simulink model "ES320A_MotDrvDiagc"  (R2013b)
settings: Solver=FixedStepDiscrete  StartTime=0.0  StopTime=1  FixedStep=.002  RelTol=1e-3
undefined symbols (not defined in the file): ARCHGLBPRM_2MILLISEC_SEC_F32, MotDrvDiagcErrFilFrq, MotDrvDiagcErrOffs, MotDrvDiagcErrThd, NtcNr1, NtcSts1, PHAONTISUMMAX_NANOSEC_U32, SysSt1
libraries: simulink x23, Fil x12, NxtrAbslt x6, NxtrLim x6
(part 3 of 3)

== system ES320A_MotDrvDiagc/MotDrvDiagc/MotDrvDiagcPer1/MotDrvDiagcFltChk/MeasdPhaFltChkABC/NtcStInfoPhaC/DetermineBitsetC1 ==
  Action Port : ActionPort  ActionType=else
  Constant5 : Constant  Value=0  OutDataTypeStr=uint8
  Copyright1 : Subsystem  Description=|  RequirementInfo={} %GIDa_4733e405_2a62_4416_a20f_f2380524059e  mask(Copyright Information){none=on}
      | Copyright info block.                                               
      |                                                                     
      | Place copyright information at the top of every subsystem in design.
      mask prompts: none "No parameters"
      mask help: Place copyright information at the top of every subsystem in design.
      mask Display:
      | NxtrConf = 'Nexteer Confidential';
      | 
      | sys = bdroot; %handle for the current model ("system")
      | first = get_param(sys,'Created');
      | if(isempty(first))
      |     first = datestr(now,'yyyy');
      | else
      |     first = first(end-3:end);  %year is last four digits
      | end
      | 
      | last = get_param(sys,'LastModifiedDate');
      | if isempty(last)
      |     last = datestr(now,'yyyy');
      | else
      |     last = last(end-3:end);
      | end
      | 
      | if strcmp(first,last)
      |     fprintf('%s\nCopyright  %s Nexteer',NxtrConf,first);
      | else
      |     fprintf('%s\n%s%s-%s Nexteer',NxtrConf,char(169),first,last);
      | end
  BitSetC : Outport
  wires:
  Constant5/1 -> BitSetC/1

== system ES320A_MotDrvDiagc/MotDrvDiagc/MotDrvDiagcPer1/MotDrvDiagcFltChk/MeasdPhaFltChkABC/NtcStsPhaABC/Copyright1 ==

== system ES320A_MotDrvDiagc/MotDrvDiagc/MotDrvDiagcPer1/MotDrvDiagcFltChk/MeasdPhaFltChkABC/NtcStsPhaABC/NtcFailed ==
  Action Port : ActionPort  ActionType=else
  Copyright1 : Subsystem  Description=|  RequirementInfo={} %GIDa_bd5e996a_5d08_43f2_9ecd_b972bb3ae5f6  mask(Copyright Information){none=on}
      | Copyright info block.                                               
      |                                                                     
      | Place copyright information at the top of every subsystem in design.
      mask prompts: none "No parameters"
      mask help: Place copyright information at the top of every subsystem in design.
      mask Display:
      | NxtrConf = 'Nexteer Confidential';
      | 
      | sys = bdroot; %handle for the current model ("system")
      | first = get_param(sys,'Created');
      | if(isempty(first))
      |     first = datestr(now,'yyyy');
      | else
      |     first = first(end-3:end);  %year is last four digits
      | end
      | 
      | last = get_param(sys,'LastModifiedDate');
      | if isempty(last)
      |     last = datestr(now,'yyyy');
      | else
      |     last = last(end-3:end);
      | end
      | 
      | if strcmp(first,last)
      |     fprintf('%s\nCopyright  %s Nexteer',NxtrConf,first);
      | else
      |     fprintf('%s\n%s%s-%s Nexteer',NxtrConf,char(169),first,last);
      | end
  NtcSts : simulink/Sources/Enumerated Constant  OutDataTypeStr=Enum: NtcSts1  Value=NtcSts1.NTCSTS_FAILD  SampleTime=inf
  NtcSts1 : Outport
  wires:
  NtcSts/1 -> NtcSts1/1

== system ES320A_MotDrvDiagc/MotDrvDiagc/MotDrvDiagcPer1/MotDrvDiagcFltChk/MeasdPhaFltChkABC/NtcStsPhaABC/NtcPassed ==
  Action Port : ActionPort  ActionType=then
  Copyright1 : Subsystem  Description=|  RequirementInfo={} %GIDa_99e6e5b4_d746_41cc_912e_5ec491f39e50  mask(Copyright Information){none=on}
      | Copyright info block.                                               
      |                                                                     
      | Place copyright information at the top of every subsystem in design.
      mask prompts: none "No parameters"
      mask help: Place copyright information at the top of every subsystem in design.
      mask Display:
      | NxtrConf = 'Nexteer Confidential';
      | 
      | sys = bdroot; %handle for the current model ("system")
      | first = get_param(sys,'Created');
      | if(isempty(first))
      |     first = datestr(now,'yyyy');
      | else
      |     first = first(end-3:end);  %year is last four digits
      | end
      | 
      | last = get_param(sys,'LastModifiedDate');
      | if isempty(last)
      |     last = datestr(now,'yyyy');
      | else
      |     last = last(end-3:end);
      | end
      | 
      | if strcmp(first,last)
      |     fprintf('%s\nCopyright  %s Nexteer',NxtrConf,first);
      | else
      |     fprintf('%s\n%s%s-%s Nexteer',NxtrConf,char(169),first,last);
      | end
  NtcSts : simulink/Sources/Enumerated Constant  OutDataTypeStr=Enum: NtcSts1  Value=NtcSts1.NTCSTS_PASSD  SampleTime=inf
  NtcSts1 : Outport
  wires:
  NtcSts/1 -> NtcSts1/1

== system ES320A_MotDrvDiagc/MotDrvDiagc/MotDrvDiagcPer1/MotDrvDiagcFltChk/MeasdPhaFltChkABC/SetNtcSts/Copyright1 ==

== system ES320A_MotDrvDiagc/MotDrvDiagc/MotDrvDiagcPer1/MotDrvDiagcFltChk/MeasdPhaFltChkDEF/FltLmtA/Copyright1 ==

== system ES320A_MotDrvDiagc/MotDrvDiagc/MotDrvDiagcPer1/MotDrvDiagcFltChk/MeasdPhaFltChkDEF/FltLmtB/Copyright1 ==

== system ES320A_MotDrvDiagc/MotDrvDiagc/MotDrvDiagcPer1/MotDrvDiagcFltChk/MeasdPhaFltChkDEF/FltLmtC/Copyright1 ==

== system ES320A_MotDrvDiagc/MotDrvDiagc/MotDrvDiagcPer1/MotDrvDiagcFltChk/MeasdPhaFltChkDEF/NtcStInfoPhaD/Copyright1 ==

== system ES320A_MotDrvDiagc/MotDrvDiagc/MotDrvDiagcPer1/MotDrvDiagcFltChk/MeasdPhaFltChkDEF/NtcStInfoPhaD/DetermineBitsetD ==
  PhaOnTiMeasdD : Inport
  PhaOnTiSumAExp : Inport  Port=2
  Action Port : ActionPort  ActionType=then
  BitsetStsD : Subsystem  RequirementInfo={'linktype_rmi_doors' '0000cf4c (/ESG Group/FDD Module Requirements/EA4 Specific/ES320A_MotDrvDiagc)' '#ES320A_196' 'true' 'REQ: ES320A_196' '' } %GIDa_8260d35a_8abd_420d_bbec_6159932b305c  TreatAsAtomicUnit=on
  BitsetStsD1 : Subsystem  RequirementInfo={'linktype_rmi_doors' '0000cf4c (/ESG Group/FDD Module Requirements/EA4 Specific/ES320A_MotDrvDiagc)' '#ES320A_197' 'true' 'REQ: ES320A_197' '' } %GIDa_48a41a6a_6f15_404d_a5f0_60e64f87e767  TreatAsAtomicUnit=on
  Copyright1 : Subsystem  Description=|  RequirementInfo={} %GIDa_1788af49_bd75_4060_896f_185cb50ec618  mask(Copyright Information){none=on}
      | Copyright info block.                                               
      |                                                                     
      | Place copyright information at the top of every subsystem in design.
      mask prompts: none "No parameters"
      mask help: Place copyright information at the top of every subsystem in design.
      mask Display:
      | NxtrConf = 'Nexteer Confidential';
      | 
      | sys = bdroot; %handle for the current model ("system")
      | first = get_param(sys,'Created');
      | if(isempty(first))
      |     first = datestr(now,'yyyy');
      | else
      |     first = first(end-3:end);  %year is last four digits
      | end
      | 
      | last = get_param(sys,'LastModifiedDate');
      | if isempty(last)
      |     last = datestr(now,'yyyy');
      | else
      |     last = last(end-3:end);
      | end
      | 
      | if strcmp(first,last)
      |     fprintf('%s\nCopyright  %s Nexteer',NxtrConf,first);
      | else
      |     fprintf('%s\n%s%s-%s Nexteer',NxtrConf,char(169),first,last);
      | end
  If : If  IfExpression=u1
  Merge : Merge
  Relational Operator : RelationalOperator  Operator=<  OutDataTypeStr=boolean
  BitSetD : Outport
  wires:
  BitsetStsD/1(bitsetD) -> Merge/1
  BitsetStsD1/1(bitsetD) -> Merge/2
  Merge/1 -> BitSetD/1
  If/1 -> BitsetStsD/Action
  PhaOnTiMeasdD/1 -> Relational Operator/1
  PhaOnTiSumAExp/1 -> Relational Operator/2
  If/2 -> BitsetStsD1/Action
  Relational Operator/1 -> If/1

== system ES320A_MotDrvDiagc/MotDrvDiagc/MotDrvDiagcPer1/MotDrvDiagcFltChk/MeasdPhaFltChkDEF/NtcStInfoPhaD/DetermineBitsetD1 ==
  Action Port : ActionPort  ActionType=else
  Constant5 : Constant  Value=0  OutDataTypeStr=uint8
  Copyright1 : Subsystem  Description=|  RequirementInfo={} %GIDa_7d3de8bf_4d93_4aaf_a970_cfd48355e2a0  mask(Copyright Information){none=on}
      | Copyright info block.                                               
      |                                                                     
      | Place copyright information at the top of every subsystem in design.
      mask prompts: none "No parameters"
      mask help: Place copyright information at the top of every subsystem in design.
      mask Display:
      | NxtrConf = 'Nexteer Confidential';
      | 
      | sys = bdroot; %handle for the current model ("system")
      | first = get_param(sys,'Created');
      | if(isempty(first))
      |     first = datestr(now,'yyyy');
      | else
      |     first = first(end-3:end);  %year is last four digits
      | end
      | 
      | last = get_param(sys,'LastModifiedDate');
      | if isempty(last)
      |     last = datestr(now,'yyyy');
      | else
      |     last = last(end-3:end);
      | end
      | 
      | if strcmp(first,last)
      |     fprintf('%s\nCopyright  %s Nexteer',NxtrConf,first);
      | else
      |     fprintf('%s\n%s%s-%s Nexteer',NxtrConf,char(169),first,last);
      | end
  BitSetD : Outport
  wires:
  Constant5/1 -> BitSetD/1

== system ES320A_MotDrvDiagc/MotDrvDiagc/MotDrvDiagcPer1/MotDrvDiagcFltChk/MeasdPhaFltChkDEF/NtcStInfoPhaE/Copyright1 ==

== system ES320A_MotDrvDiagc/MotDrvDiagc/MotDrvDiagcPer1/MotDrvDiagcFltChk/MeasdPhaFltChkDEF/NtcStInfoPhaE/DetermineBitsetE ==
  PhaOnTiMeasdE : Inport
  PhaOnTiSumBExp : Inport  Port=2
  Action Port : ActionPort  ActionType=then
  BitsetStsE : Subsystem  RequirementInfo={'linktype_rmi_doors' '0000cf4c (/ESG Group/FDD Module Requirements/EA4 Specific/ES320A_MotDrvDiagc)' '#ES320A_198' 'true' 'REQ: ES320A_198' '' } %GIDa_08169722_133b_47d0_8dcc_55ebdb8fb1a5  TreatAsAtomicUnit=on
  BitsetStsE1 : Subsystem  RequirementInfo={'linktype_rmi_doors' '0000cf4c (/ESG Group/FDD Module Requirements/EA4 Specific/ES320A_MotDrvDiagc)' '#ES320A_199' 'true' 'REQ: ES320A_199' '' } %GIDa_359415b0_e38b_416f_8765_3117a83da501  TreatAsAtomicUnit=on
  Copyright1 : Subsystem  Description=|  RequirementInfo={} %GIDa_7c5a11b8_a3a6_4c1e_aad7_eeec68a14235  mask(Copyright Information){none=on}
      | Copyright info block.                                               
      |                                                                     
      | Place copyright information at the top of every subsystem in design.
      mask prompts: none "No parameters"
      mask help: Place copyright information at the top of every subsystem in design.
      mask Display:
      | NxtrConf = 'Nexteer Confidential';
      | 
      | sys = bdroot; %handle for the current model ("system")
      | first = get_param(sys,'Created');
      | if(isempty(first))
      |     first = datestr(now,'yyyy');
      | else
      |     first = first(end-3:end);  %year is last four digits
      | end
      | 
      | last = get_param(sys,'LastModifiedDate');
      | if isempty(last)
      |     last = datestr(now,'yyyy');
      | else
      |     last = last(end-3:end);
      | end
      | 
      | if strcmp(first,last)
      |     fprintf('%s\nCopyright  %s Nexteer',NxtrConf,first);
      | else
      |     fprintf('%s\n%s%s-%s Nexteer',NxtrConf,char(169),first,last);
      | end
  If : If  IfExpression=u1
  Merge : Merge
  Relational Operator : RelationalOperator  Operator=<  OutDataTypeStr=boolean
  BitSetE : Outport
  wires:
  PhaOnTiSumBExp/1 -> Relational Operator/2
  PhaOnTiMeasdE/1 -> Relational Operator/1
  BitsetStsE/1(bitsetE) -> Merge/1
  BitsetStsE1/1(bitsetE) -> Merge/2
  Merge/1 -> BitSetE/1
  If/1 -> BitsetStsE/Action
  If/2 -> BitsetStsE1/Action
  Relational Operator/1 -> If/1

== system ES320A_MotDrvDiagc/MotDrvDiagc/MotDrvDiagcPer1/MotDrvDiagcFltChk/MeasdPhaFltChkDEF/NtcStInfoPhaE/DetermineBitsetE1 ==
  Action Port : ActionPort  ActionType=else
  Constant5 : Constant  Value=0  OutDataTypeStr=uint8
  Copyright1 : Subsystem  Description=|  RequirementInfo={} %GIDa_2e7c738b_8ed4_4057_8dbe_cf0f29a374b5  mask(Copyright Information){none=on}
      | Copyright info block.                                               
      |                                                                     
      | Place copyright information at the top of every subsystem in design.
      mask prompts: none "No parameters"
      mask help: Place copyright information at the top of every subsystem in design.
      mask Display:
      | NxtrConf = 'Nexteer Confidential';
      | 
      | sys = bdroot; %handle for the current model ("system")
      | first = get_param(sys,'Created');
      | if(isempty(first))
      |     first = datestr(now,'yyyy');
      | else
      |     first = first(end-3:end);  %year is last four digits
      | end
      | 
      | last = get_param(sys,'LastModifiedDate');
      | if isempty(last)
      |     last = datestr(now,'yyyy');
      | else
      |     last = last(end-3:end);
      | end
      | 
      | if strcmp(first,last)
      |     fprintf('%s\nCopyright  %s Nexteer',NxtrConf,first);
      | else
      |     fprintf('%s\n%s%s-%s Nexteer',NxtrConf,char(169),first,last);
      | end
  BitSetE : Outport
  wires:
  Constant5/1 -> BitSetE/1

== system ES320A_MotDrvDiagc/MotDrvDiagc/MotDrvDiagcPer1/MotDrvDiagcFltChk/MeasdPhaFltChkDEF/NtcStInfoPhaF/Copyright1 ==

== system ES320A_MotDrvDiagc/MotDrvDiagc/MotDrvDiagcPer1/MotDrvDiagcFltChk/MeasdPhaFltChkDEF/NtcStInfoPhaF/DetermineBitsetF ==
  PhaOnTiMeasdF : Inport
  PhaOnTiSumCExp : Inport  Port=2
  Action Port : ActionPort  ActionType=then
  BitsetStsF : Subsystem  RequirementInfo={'linktype_rmi_doors' '0000cf4c (/ESG Group/FDD Module Requirements/EA4 Specific/ES320A_MotDrvDiagc)' '#ES320A_200' 'true' 'REQ: ES320A_200' '' } %GIDa_55a58c0c_abfb_4587_b479_1d90e8aa5549  TreatAsAtomicUnit=on
  BitsetStsF1 : Subsystem  RequirementInfo={'linktype_rmi_doors' '0000cf4c (/ESG Group/FDD Module Requirements/EA4 Specific/ES320A_MotDrvDiagc)' '#ES320A_201' 'true' 'REQ: ES320A_201' '' } %GIDa_a8dfb83c_85c1_4b48_a1e1_aa37e2bdfe1a  TreatAsAtomicUnit=on
  Copyright1 : Subsystem  Description=|  RequirementInfo={} %GIDa_fb0ae897_2b05_462f_9fe8_c1b0d422596f  mask(Copyright Information){none=on}
      | Copyright info block.                                               
      |                                                                     
      | Place copyright information at the top of every subsystem in design.
      mask prompts: none "No parameters"
      mask help: Place copyright information at the top of every subsystem in design.
      mask Display:
      | NxtrConf = 'Nexteer Confidential';
      | 
      | sys = bdroot; %handle for the current model ("system")
      | first = get_param(sys,'Created');
      | if(isempty(first))
      |     first = datestr(now,'yyyy');
      | else
      |     first = first(end-3:end);  %year is last four digits
      | end
      | 
      | last = get_param(sys,'LastModifiedDate');
      | if isempty(last)
      |     last = datestr(now,'yyyy');
      | else
      |     last = last(end-3:end);
      | end
      | 
      | if strcmp(first,last)
      |     fprintf('%s\nCopyright  %s Nexteer',NxtrConf,first);
      | else
      |     fprintf('%s\n%s%s-%s Nexteer',NxtrConf,char(169),first,last);
      | end
  If : If  IfExpression=u1
  Merge : Merge
  Relational Operator : RelationalOperator  Operator=<  OutDataTypeStr=boolean
  BitSetF : Outport
  wires:
  BitsetStsF/1(bitsetF) -> Merge/1
  BitsetStsF1/1(bitsetF) -> Merge/2
  Merge/1 -> BitSetF/1
  PhaOnTiSumCExp/1 -> Relational Operator/2
  PhaOnTiMeasdF/1 -> Relational Operator/1
  If/1 -> BitsetStsF/Action
  If/2 -> BitsetStsF1/Action
  Relational Operator/1 -> If/1

== system ES320A_MotDrvDiagc/MotDrvDiagc/MotDrvDiagcPer1/MotDrvDiagcFltChk/MeasdPhaFltChkDEF/NtcStInfoPhaF/DetermineBitsetF1 ==
  Action Port : ActionPort  ActionType=else
  Constant5 : Constant  Value=0  OutDataTypeStr=uint8
  Copyright1 : Subsystem  Description=|  RequirementInfo={} %GIDa_d82a1e1b_c682_4f73_a346_e773759e2be9  mask(Copyright Information){none=on}
      | Copyright info block.                                               
      |                                                                     
      | Place copyright information at the top of every subsystem in design.
      mask prompts: none "No parameters"
      mask help: Place copyright information at the top of every subsystem in design.
      mask Display:
      | NxtrConf = 'Nexteer Confidential';
      | 
      | sys = bdroot; %handle for the current model ("system")
      | first = get_param(sys,'Created');
      | if(isempty(first))
      |     first = datestr(now,'yyyy');
      | else
      |     first = first(end-3:end);  %year is last four digits
      | end
      | 
      | last = get_param(sys,'LastModifiedDate');
      | if isempty(last)
      |     last = datestr(now,'yyyy');
      | else
      |     last = last(end-3:end);
      | end
      | 
      | if strcmp(first,last)
      |     fprintf('%s\nCopyright  %s Nexteer',NxtrConf,first);
      | else
      |     fprintf('%s\n%s%s-%s Nexteer',NxtrConf,char(169),first,last);
      | end
  BitSetF : Outport
  wires:
  Constant5/1 -> BitSetF/1

== system ES320A_MotDrvDiagc/MotDrvDiagc/MotDrvDiagcPer1/MotDrvDiagcFltChk/MeasdPhaFltChkDEF/NtcStsPhaDEF/Copyright1 ==

== system ES320A_MotDrvDiagc/MotDrvDiagc/MotDrvDiagcPer1/MotDrvDiagcFltChk/MeasdPhaFltChkDEF/NtcStsPhaDEF/NtcFailed ==
  Action Port : ActionPort  ActionType=else
  Copyright1 : Subsystem  Description=|  RequirementInfo={} %GIDa_17e947be_2e1f_4709_9ef4_8520ceffa1b1  mask(Copyright Information){none=on}
      | Copyright info block.                                               
      |                                                                     
      | Place copyright information at the top of every subsystem in design.
      mask prompts: none "No parameters"
      mask help: Place copyright information at the top of every subsystem in design.
      mask Display:
      | NxtrConf = 'Nexteer Confidential';
      | 
      | sys = bdroot; %handle for the current model ("system")
      | first = get_param(sys,'Created');
      | if(isempty(first))
      |     first = datestr(now,'yyyy');
      | else
      |     first = first(end-3:end);  %year is last four digits
      | end
      | 
      | last = get_param(sys,'LastModifiedDate');
      | if isempty(last)
      |     last = datestr(now,'yyyy');
      | else
      |     last = last(end-3:end);
      | end
      | 
      | if strcmp(first,last)
      |     fprintf('%s\nCopyright  %s Nexteer',NxtrConf,first);
      | else
      |     fprintf('%s\n%s%s-%s Nexteer',NxtrConf,char(169),first,last);
      | end
  NtcSts : simulink/Sources/Enumerated Constant  OutDataTypeStr=Enum: NtcSts1  Value=NtcSts1.NTCSTS_FAILD  SampleTime=inf
  NtcSts1 : Outport
  wires:
  NtcSts/1 -> NtcSts1/1

== system ES320A_MotDrvDiagc/MotDrvDiagc/MotDrvDiagcPer1/MotDrvDiagcFltChk/MeasdPhaFltChkDEF/NtcStsPhaDEF/NtcPassed ==
  Action Port : ActionPort  ActionType=then
  Copyright1 : Subsystem  Description=|  RequirementInfo={} %GIDa_1122f953_822e_40b1_bb4c_1cb6bb86ea20  mask(Copyright Information){none=on}
      | Copyright info block.                                               
      |                                                                     
      | Place copyright information at the top of every subsystem in design.
      mask prompts: none "No parameters"
      mask help: Place copyright information at the top of every subsystem in design.
      mask Display:
      | NxtrConf = 'Nexteer Confidential';
      | 
      | sys = bdroot; %handle for the current model ("system")
      | first = get_param(sys,'Created');
      | if(isempty(first))
      |     first = datestr(now,'yyyy');
      | else
      |     first = first(end-3:end);  %year is last four digits
      | end
      | 
      | last = get_param(sys,'LastModifiedDate');
      | if isempty(last)
      |     last = datestr(now,'yyyy');
      | else
      |     last = last(end-3:end);
      | end
      | 
      | if strcmp(first,last)
      |     fprintf('%s\nCopyright  %s Nexteer',NxtrConf,first);
      | else
      |     fprintf('%s\n%s%s-%s Nexteer',NxtrConf,char(169),first,last);
      | end
  NtcSts : simulink/Sources/Enumerated Constant  OutDataTypeStr=Enum: NtcSts1  Value=NtcSts1.NTCSTS_PASSD  SampleTime=inf
  NtcSts1 : Outport
  wires:
  NtcSts/1 -> NtcSts1/1

== system ES320A_MotDrvDiagc/MotDrvDiagc/MotDrvDiagcPer1/MotDrvDiagcFltChk/MeasdPhaFltChkDEF/SetNtcSts/Copyright1 ==

== system ES320A_MotDrvDiagc/MotDrvDiagc/MotDrvDiagcPer1/MotDrvDiagcFltChk/MeasdPhaFltChkABC/NtcStInfoPhaA/DetermineBitsetA/BitsetStsA ==
  Action Port : ActionPort  ActionType=then
  Bit Set : simulink/Logic and Bit Operations/Bit Set  iBit=0
  Constant : Constant  Value=0  OutDataTypeStr=uint8
  Copyright1 : Subsystem  Description=|  RequirementInfo={} %GIDa_cdd52c65_1ab2_45c6_a6fc_5222191c335e  mask(Copyright Information){none=on}
      | Copyright info block.                                               
      |                                                                     
      | Place copyright information at the top of every subsystem in design.
      mask prompts: none "No parameters"
      mask help: Place copyright information at the top of every subsystem in design.
      mask Display:
      | NxtrConf = 'Nexteer Confidential';
      | 
      | sys = bdroot; %handle for the current model ("system")
      | first = get_param(sys,'Created');
      | if(isempty(first))
      |     first = datestr(now,'yyyy');
      | else
      |     first = first(end-3:end);  %year is last four digits
      | end
      | 
      | last = get_param(sys,'LastModifiedDate');
      | if isempty(last)
      |     last = datestr(now,'yyyy');
      | else
      |     last = last(end-3:end);
      | end
      | 
      | if strcmp(first,last)
      |     fprintf('%s\nCopyright  %s Nexteer',NxtrConf,first);
      | else
      |     fprintf('%s\n%s%s-%s Nexteer',NxtrConf,char(169),first,last);
      | end
  bitsetA : Outport
  wires:
  Constant/1 -> Bit Set/1
  Bit Set/1 -> bitsetA/1

== system ES320A_MotDrvDiagc/MotDrvDiagc/MotDrvDiagcPer1/MotDrvDiagcFltChk/MeasdPhaFltChkABC/NtcStInfoPhaA/DetermineBitsetA/BitsetStsA1 ==
  Action Port : ActionPort  ActionType=else
  Bit Set1 : simulink/Logic and Bit Operations/Bit Set  iBit=1
  Constant6 : Constant  Value=0  OutDataTypeStr=uint8
  Copyright1 : Subsystem  Description=|  RequirementInfo={} %GIDa_4a3532e0_542b_44ef_af96_af0d103a28d1  mask(Copyright Information){none=on}
      | Copyright info block.                                               
      |                                                                     
      | Place copyright information at the top of every subsystem in design.
      mask prompts: none "No parameters"
      mask help: Place copyright information at the top of every subsystem in design.
      mask Display:
      | NxtrConf = 'Nexteer Confidential';
      | 
      | sys = bdroot; %handle for the current model ("system")
      | first = get_param(sys,'Created');
      | if(isempty(first))
      |     first = datestr(now,'yyyy');
      | else
      |     first = first(end-3:end);  %year is last four digits
      | end
      | 
      | last = get_param(sys,'LastModifiedDate');
      | if isempty(last)
      |     last = datestr(now,'yyyy');
      | else
      |     last = last(end-3:end);
      | end
      | 
      | if strcmp(first,last)
      |     fprintf('%s\nCopyright  %s Nexteer',NxtrConf,first);
      | else
      |     fprintf('%s\n%s%s-%s Nexteer',NxtrConf,char(169),first,last);
      | end
  bitsetA : Outport
  wires:
  Constant6/1 -> Bit Set1/1
  Bit Set1/1 -> bitsetA/1

== system ES320A_MotDrvDiagc/MotDrvDiagc/MotDrvDiagcPer1/MotDrvDiagcFltChk/MeasdPhaFltChkABC/NtcStInfoPhaA/DetermineBitsetA/Copyright1 ==

== system ES320A_MotDrvDiagc/MotDrvDiagc/MotDrvDiagcPer1/MotDrvDiagcFltChk/MeasdPhaFltChkABC/NtcStInfoPhaA/DetermineBitsetA1/Copyright1 ==

== system ES320A_MotDrvDiagc/MotDrvDiagc/MotDrvDiagcPer1/MotDrvDiagcFltChk/MeasdPhaFltChkABC/NtcStInfoPhaB/DetermineBitsetB/BitsetStsB ==
  Action Port : ActionPort  ActionType=then
  Bit Set : simulink/Logic and Bit Operations/Bit Set  iBit=2
  Constant : Constant  Value=0  OutDataTypeStr=uint8
  Copyright1 : Subsystem  Description=|  RequirementInfo={} %GIDa_c1b71190_810a_4c1f_9336_9d9ddd65ac32  mask(Copyright Information){none=on}
      | Copyright info block.                                               
      |                                                                     
      | Place copyright information at the top of every subsystem in design.
      mask prompts: none "No parameters"
      mask help: Place copyright information at the top of every subsystem in design.
      mask Display:
      | NxtrConf = 'Nexteer Confidential';
      | 
      | sys = bdroot; %handle for the current model ("system")
      | first = get_param(sys,'Created');
      | if(isempty(first))
      |     first = datestr(now,'yyyy');
      | else
      |     first = first(end-3:end);  %year is last four digits
      | end
      | 
      | last = get_param(sys,'LastModifiedDate');
      | if isempty(last)
      |     last = datestr(now,'yyyy');
      | else
      |     last = last(end-3:end);
      | end
      | 
      | if strcmp(first,last)
      |     fprintf('%s\nCopyright  %s Nexteer',NxtrConf,first);
      | else
      |     fprintf('%s\n%s%s-%s Nexteer',NxtrConf,char(169),first,last);
      | end
  bitsetB : Outport
  wires:
  Constant/1 -> Bit Set/1
  Bit Set/1 -> bitsetB/1

== system ES320A_MotDrvDiagc/MotDrvDiagc/MotDrvDiagcPer1/MotDrvDiagcFltChk/MeasdPhaFltChkABC/NtcStInfoPhaB/DetermineBitsetB/BitsetStsB1 ==
  Action Port : ActionPort  ActionType=else
  Bit Set1 : simulink/Logic and Bit Operations/Bit Set  iBit=3
  Constant6 : Constant  Value=0  OutDataTypeStr=uint8
  Copyright1 : Subsystem  Description=|  RequirementInfo={} %GIDa_1c98625e_4ddf_4d14_b0b0_5f8b66934288  mask(Copyright Information){none=on}
      | Copyright info block.                                               
      |                                                                     
      | Place copyright information at the top of every subsystem in design.
      mask prompts: none "No parameters"
      mask help: Place copyright information at the top of every subsystem in design.
      mask Display:
      | NxtrConf = 'Nexteer Confidential';
      | 
      | sys = bdroot; %handle for the current model ("system")
      | first = get_param(sys,'Created');
      | if(isempty(first))
      |     first = datestr(now,'yyyy');
      | else
      |     first = first(end-3:end);  %year is last four digits
      | end
      | 
      | last = get_param(sys,'LastModifiedDate');
      | if isempty(last)
      |     last = datestr(now,'yyyy');
      | else
      |     last = last(end-3:end);
      | end
      | 
      | if strcmp(first,last)
      |     fprintf('%s\nCopyright  %s Nexteer',NxtrConf,first);
      | else
      |     fprintf('%s\n%s%s-%s Nexteer',NxtrConf,char(169),first,last);
      | end
  bitsetB : Outport
  wires:
  Constant6/1 -> Bit Set1/1
  Bit Set1/1 -> bitsetB/1

== system ES320A_MotDrvDiagc/MotDrvDiagc/MotDrvDiagcPer1/MotDrvDiagcFltChk/MeasdPhaFltChkABC/NtcStInfoPhaB/DetermineBitsetB/Copyright1 ==

== system ES320A_MotDrvDiagc/MotDrvDiagc/MotDrvDiagcPer1/MotDrvDiagcFltChk/MeasdPhaFltChkABC/NtcStInfoPhaB/DetermineBitsetB1/Copyright1 ==

== system ES320A_MotDrvDiagc/MotDrvDiagc/MotDrvDiagcPer1/MotDrvDiagcFltChk/MeasdPhaFltChkABC/NtcStInfoPhaC/DetermineBitsetC/BitsetStsC ==
  Action Port : ActionPort  ActionType=then
  Bit Set : simulink/Logic and Bit Operations/Bit Set  iBit=4
  Constant : Constant  Value=0  OutDataTypeStr=uint8
  Copyright1 : Subsystem  Description=|  RequirementInfo={} %GIDa_c7f9e4bd_06f8_4d47_b8c3_bba4ebe2b271  mask(Copyright Information){none=on}
      | Copyright info block.                                               
      |                                                                     
      | Place copyright information at the top of every subsystem in design.
      mask prompts: none "No parameters"
      mask help: Place copyright information at the top of every subsystem in design.
      mask Display:
      | NxtrConf = 'Nexteer Confidential';
      | 
      | sys = bdroot; %handle for the current model ("system")
      | first = get_param(sys,'Created');
      | if(isempty(first))
      |     first = datestr(now,'yyyy');
      | else
      |     first = first(end-3:end);  %year is last four digits
      | end
      | 
      | last = get_param(sys,'LastModifiedDate');
      | if isempty(last)
      |     last = datestr(now,'yyyy');
      | else
      |     last = last(end-3:end);
      | end
      | 
      | if strcmp(first,last)
      |     fprintf('%s\nCopyright  %s Nexteer',NxtrConf,first);
      | else
      |     fprintf('%s\n%s%s-%s Nexteer',NxtrConf,char(169),first,last);
      | end
  bitsetC : Outport
  wires:
  Constant/1 -> Bit Set/1
  Bit Set/1 -> bitsetC/1

== system ES320A_MotDrvDiagc/MotDrvDiagc/MotDrvDiagcPer1/MotDrvDiagcFltChk/MeasdPhaFltChkABC/NtcStInfoPhaC/DetermineBitsetC/BitsetStsC1 ==
  Action Port : ActionPort  ActionType=else
  Bit Set1 : simulink/Logic and Bit Operations/Bit Set  iBit=5
  Constant6 : Constant  Value=0  OutDataTypeStr=uint8
  Copyright1 : Subsystem  Description=|  RequirementInfo={} %GIDa_6c0cda01_92a0_4b9b_997e_e6f0ddc1bb0d  mask(Copyright Information){none=on}
      | Copyright info block.                                               
      |                                                                     
      | Place copyright information at the top of every subsystem in design.
      mask prompts: none "No parameters"
      mask help: Place copyright information at the top of every subsystem in design.
      mask Display:
      | NxtrConf = 'Nexteer Confidential';
      | 
      | sys = bdroot; %handle for the current model ("system")
      | first = get_param(sys,'Created');
      | if(isempty(first))
      |     first = datestr(now,'yyyy');
      | else
      |     first = first(end-3:end);  %year is last four digits
      | end
      | 
      | last = get_param(sys,'LastModifiedDate');
      | if isempty(last)
      |     last = datestr(now,'yyyy');
      | else
      |     last = last(end-3:end);
      | end
      | 
      | if strcmp(first,last)
      |     fprintf('%s\nCopyright  %s Nexteer',NxtrConf,first);
      | else
      |     fprintf('%s\n%s%s-%s Nexteer',NxtrConf,char(169),first,last);
      | end
  bitsetC : Outport
  wires:
  Constant6/1 -> Bit Set1/1
  Bit Set1/1 -> bitsetC/1

== system ES320A_MotDrvDiagc/MotDrvDiagc/MotDrvDiagcPer1/MotDrvDiagcFltChk/MeasdPhaFltChkABC/NtcStInfoPhaC/DetermineBitsetC/Copyright1 ==

== system ES320A_MotDrvDiagc/MotDrvDiagc/MotDrvDiagcPer1/MotDrvDiagcFltChk/MeasdPhaFltChkABC/NtcStInfoPhaC/DetermineBitsetC1/Copyright1 ==

== system ES320A_MotDrvDiagc/MotDrvDiagc/MotDrvDiagcPer1/MotDrvDiagcFltChk/MeasdPhaFltChkABC/NtcStsPhaABC/NtcFailed/Copyright1 ==

== system ES320A_MotDrvDiagc/MotDrvDiagc/MotDrvDiagcPer1/MotDrvDiagcFltChk/MeasdPhaFltChkABC/NtcStsPhaABC/NtcPassed/Copyright1 ==

== system ES320A_MotDrvDiagc/MotDrvDiagc/MotDrvDiagcPer1/MotDrvDiagcFltChk/MeasdPhaFltChkDEF/NtcStInfoPhaD/DetermineBitsetD/BitsetStsD ==
  Action Port : ActionPort  ActionType=then
  Bit Set : simulink/Logic and Bit Operations/Bit Set  iBit=0
  Constant : Constant  Value=0  OutDataTypeStr=uint8
  Copyright1 : Subsystem  Description=|  RequirementInfo={} %GIDa_dbcf2c0d_978d_4fef_ba7e_03b850f9e23e  mask(Copyright Information){none=on}
      | Copyright info block.                                               
      |                                                                     
      | Place copyright information at the top of every subsystem in design.
      mask prompts: none "No parameters"
      mask help: Place copyright information at the top of every subsystem in design.
      mask Display:
      | NxtrConf = 'Nexteer Confidential';
      | 
      | sys = bdroot; %handle for the current model ("system")
      | first = get_param(sys,'Created');
      | if(isempty(first))
      |     first = datestr(now,'yyyy');
      | else
      |     first = first(end-3:end);  %year is last four digits
      | end
      | 
      | last = get_param(sys,'LastModifiedDate');
      | if isempty(last)
      |     last = datestr(now,'yyyy');
      | else
      |     last = last(end-3:end);
      | end
      | 
      | if strcmp(first,last)
      |     fprintf('%s\nCopyright  %s Nexteer',NxtrConf,first);
      | else
      |     fprintf('%s\n%s%s-%s Nexteer',NxtrConf,char(169),first,last);
      | end
  bitsetD : Outport
  wires:
  Constant/1 -> Bit Set/1
  Bit Set/1 -> bitsetD/1

== system ES320A_MotDrvDiagc/MotDrvDiagc/MotDrvDiagcPer1/MotDrvDiagcFltChk/MeasdPhaFltChkDEF/NtcStInfoPhaD/DetermineBitsetD/BitsetStsD1 ==
  Action Port : ActionPort  ActionType=else
  Bit Set1 : simulink/Logic and Bit Operations/Bit Set  iBit=1
  Constant6 : Constant  Value=0  OutDataTypeStr=uint8
  Copyright1 : Subsystem  Description=|  RequirementInfo={} %GIDa_acf3be0f_e4e4_4ec5_9a2d_161905b035c2  mask(Copyright Information){none=on}
      | Copyright info block.                                               
      |                                                                     
      | Place copyright information at the top of every subsystem in design.
      mask prompts: none "No parameters"
      mask help: Place copyright information at the top of every subsystem in design.
      mask Display:
      | NxtrConf = 'Nexteer Confidential';
      | 
      | sys = bdroot; %handle for the current model ("system")
      | first = get_param(sys,'Created');
      | if(isempty(first))
      |     first = datestr(now,'yyyy');
      | else
      |     first = first(end-3:end);  %year is last four digits
      | end
      | 
      | last = get_param(sys,'LastModifiedDate');
      | if isempty(last)
      |     last = datestr(now,'yyyy');
      | else
      |     last = last(end-3:end);
      | end
      | 
      | if strcmp(first,last)
      |     fprintf('%s\nCopyright  %s Nexteer',NxtrConf,first);
      | else
      |     fprintf('%s\n%s%s-%s Nexteer',NxtrConf,char(169),first,last);
      | end
  bitsetD : Outport
  wires:
  Constant6/1 -> Bit Set1/1
  Bit Set1/1 -> bitsetD/1

== system ES320A_MotDrvDiagc/MotDrvDiagc/MotDrvDiagcPer1/MotDrvDiagcFltChk/MeasdPhaFltChkDEF/NtcStInfoPhaD/DetermineBitsetD/Copyright1 ==

== system ES320A_MotDrvDiagc/MotDrvDiagc/MotDrvDiagcPer1/MotDrvDiagcFltChk/MeasdPhaFltChkDEF/NtcStInfoPhaD/DetermineBitsetD1/Copyright1 ==

== system ES320A_MotDrvDiagc/MotDrvDiagc/MotDrvDiagcPer1/MotDrvDiagcFltChk/MeasdPhaFltChkDEF/NtcStInfoPhaE/DetermineBitsetE/BitsetStsE ==
  Action Port : ActionPort  ActionType=then
  Bit Set : simulink/Logic and Bit Operations/Bit Set  iBit=2
  Constant : Constant  Value=0  OutDataTypeStr=uint8
  Copyright1 : Subsystem  Description=|  RequirementInfo={} %GIDa_171d4bfc_3d2c_4a24_aadb_9834f4df825a  mask(Copyright Information){none=on}
      | Copyright info block.                                               
      |                                                                     
      | Place copyright information at the top of every subsystem in design.
      mask prompts: none "No parameters"
      mask help: Place copyright information at the top of every subsystem in design.
      mask Display:
      | NxtrConf = 'Nexteer Confidential';
      | 
      | sys = bdroot; %handle for the current model ("system")
      | first = get_param(sys,'Created');
      | if(isempty(first))
      |     first = datestr(now,'yyyy');
      | else
      |     first = first(end-3:end);  %year is last four digits
      | end
      | 
      | last = get_param(sys,'LastModifiedDate');
      | if isempty(last)
      |     last = datestr(now,'yyyy');
      | else
      |     last = last(end-3:end);
      | end
      | 
      | if strcmp(first,last)
      |     fprintf('%s\nCopyright  %s Nexteer',NxtrConf,first);
      | else
      |     fprintf('%s\n%s%s-%s Nexteer',NxtrConf,char(169),first,last);
      | end
  bitsetE : Outport
  wires:
  Constant/1 -> Bit Set/1
  Bit Set/1 -> bitsetE/1

== system ES320A_MotDrvDiagc/MotDrvDiagc/MotDrvDiagcPer1/MotDrvDiagcFltChk/MeasdPhaFltChkDEF/NtcStInfoPhaE/DetermineBitsetE/BitsetStsE1 ==
  Action Port : ActionPort  ActionType=else
  Bit Set1 : simulink/Logic and Bit Operations/Bit Set  iBit=3
  Constant6 : Constant  Value=0  OutDataTypeStr=uint8
  Copyright1 : Subsystem  Description=|  RequirementInfo={} %GIDa_569b9211_e1ff_4771_81ec_60442d8817e2  mask(Copyright Information){none=on}
      | Copyright info block.                                               
      |                                                                     
      | Place copyright information at the top of every subsystem in design.
      mask prompts: none "No parameters"
      mask help: Place copyright information at the top of every subsystem in design.
      mask Display:
      | NxtrConf = 'Nexteer Confidential';
      | 
      | sys = bdroot; %handle for the current model ("system")
      | first = get_param(sys,'Created');
      | if(isempty(first))
      |     first = datestr(now,'yyyy');
      | else
      |     first = first(end-3:end);  %year is last four digits
      | end
      | 
      | last = get_param(sys,'LastModifiedDate');
      | if isempty(last)
      |     last = datestr(now,'yyyy');
      | else
      |     last = last(end-3:end);
      | end
      | 
      | if strcmp(first,last)
      |     fprintf('%s\nCopyright  %s Nexteer',NxtrConf,first);
      | else
      |     fprintf('%s\n%s%s-%s Nexteer',NxtrConf,char(169),first,last);
      | end
  bitsetE : Outport
  wires:
  Constant6/1 -> Bit Set1/1
  Bit Set1/1 -> bitsetE/1

== system ES320A_MotDrvDiagc/MotDrvDiagc/MotDrvDiagcPer1/MotDrvDiagcFltChk/MeasdPhaFltChkDEF/NtcStInfoPhaE/DetermineBitsetE/Copyright1 ==

== system ES320A_MotDrvDiagc/MotDrvDiagc/MotDrvDiagcPer1/MotDrvDiagcFltChk/MeasdPhaFltChkDEF/NtcStInfoPhaE/DetermineBitsetE1/Copyright1 ==

== system ES320A_MotDrvDiagc/MotDrvDiagc/MotDrvDiagcPer1/MotDrvDiagcFltChk/MeasdPhaFltChkDEF/NtcStInfoPhaF/DetermineBitsetF/BitsetStsF ==
  Action Port : ActionPort  ActionType=then
  Bit Set : simulink/Logic and Bit Operations/Bit Set  iBit=4
  Constant : Constant  Value=0  OutDataTypeStr=uint8
  Copyright1 : Subsystem  Description=|  RequirementInfo={} %GIDa_4af6ed9a_36c8_443f_b84c_44960506cf89  mask(Copyright Information){none=on}
      | Copyright info block.                                               
      |                                                                     
      | Place copyright information at the top of every subsystem in design.
      mask prompts: none "No parameters"
      mask help: Place copyright information at the top of every subsystem in design.
      mask Display:
      | NxtrConf = 'Nexteer Confidential';
      | 
      | sys = bdroot; %handle for the current model ("system")
      | first = get_param(sys,'Created');
      | if(isempty(first))
      |     first = datestr(now,'yyyy');
      | else
      |     first = first(end-3:end);  %year is last four digits
      | end
      | 
      | last = get_param(sys,'LastModifiedDate');
      | if isempty(last)
      |     last = datestr(now,'yyyy');
      | else
      |     last = last(end-3:end);
      | end
      | 
      | if strcmp(first,last)
      |     fprintf('%s\nCopyright  %s Nexteer',NxtrConf,first);
      | else
      |     fprintf('%s\n%s%s-%s Nexteer',NxtrConf,char(169),first,last);
      | end
  bitsetF : Outport
  wires:
  Constant/1 -> Bit Set/1
  Bit Set/1 -> bitsetF/1

== system ES320A_MotDrvDiagc/MotDrvDiagc/MotDrvDiagcPer1/MotDrvDiagcFltChk/MeasdPhaFltChkDEF/NtcStInfoPhaF/DetermineBitsetF/BitsetStsF1 ==
  Action Port : ActionPort  ActionType=else
  Bit Set1 : simulink/Logic and Bit Operations/Bit Set  iBit=5
  Constant6 : Constant  Value=0  OutDataTypeStr=uint8
  Copyright1 : Subsystem  Description=|  RequirementInfo={} %GIDa_7be13ad6_7ee7_4a14_98bb_dde27525f142  mask(Copyright Information){none=on}
      | Copyright info block.                                               
      |                                                                     
      | Place copyright information at the top of every subsystem in design.
      mask prompts: none "No parameters"
      mask help: Place copyright information at the top of every subsystem in design.
      mask Display:
      | NxtrConf = 'Nexteer Confidential';
      | 
      | sys = bdroot; %handle for the current model ("system")
      | first = get_param(sys,'Created');
      | if(isempty(first))
      |     first = datestr(now,'yyyy');
      | else
      |     first = first(end-3:end);  %year is last four digits
      | end
      | 
      | last = get_param(sys,'LastModifiedDate');
      | if isempty(last)
      |     last = datestr(now,'yyyy');
      | else
      |     last = last(end-3:end);
      | end
      | 
      | if strcmp(first,last)
      |     fprintf('%s\nCopyright  %s Nexteer',NxtrConf,first);
      | else
      |     fprintf('%s\n%s%s-%s Nexteer',NxtrConf,char(169),first,last);
      | end
  bitsetF : Outport
  wires:
  Constant6/1 -> Bit Set1/1
  Bit Set1/1 -> bitsetF/1

== system ES320A_MotDrvDiagc/MotDrvDiagc/MotDrvDiagcPer1/MotDrvDiagcFltChk/MeasdPhaFltChkDEF/NtcStInfoPhaF/DetermineBitsetF/Copyright1 ==

== system ES320A_MotDrvDiagc/MotDrvDiagc/MotDrvDiagcPer1/MotDrvDiagcFltChk/MeasdPhaFltChkDEF/NtcStInfoPhaF/DetermineBitsetF1/Copyright1 ==

== system ES320A_MotDrvDiagc/MotDrvDiagc/MotDrvDiagcPer1/MotDrvDiagcFltChk/MeasdPhaFltChkDEF/NtcStsPhaDEF/NtcFailed/Copyright1 ==

== system ES320A_MotDrvDiagc/MotDrvDiagc/MotDrvDiagcPer1/MotDrvDiagcFltChk/MeasdPhaFltChkDEF/NtcStsPhaDEF/NtcPassed/Copyright1 ==

== system ES320A_MotDrvDiagc/MotDrvDiagc/MotDrvDiagcPer1/MotDrvDiagcFltChk/MeasdPhaFltChkABC/NtcStInfoPhaA/DetermineBitsetA/BitsetStsA/Copyright1 ==

== system ES320A_MotDrvDiagc/MotDrvDiagc/MotDrvDiagcPer1/MotDrvDiagcFltChk/MeasdPhaFltChkABC/NtcStInfoPhaA/DetermineBitsetA/BitsetStsA1/Copyright1 ==

== system ES320A_MotDrvDiagc/MotDrvDiagc/MotDrvDiagcPer1/MotDrvDiagcFltChk/MeasdPhaFltChkABC/NtcStInfoPhaB/DetermineBitsetB/BitsetStsB/Copyright1 ==

== system ES320A_MotDrvDiagc/MotDrvDiagc/MotDrvDiagcPer1/MotDrvDiagcFltChk/MeasdPhaFltChkABC/NtcStInfoPhaB/DetermineBitsetB/BitsetStsB1/Copyright1 ==

== system ES320A_MotDrvDiagc/MotDrvDiagc/MotDrvDiagcPer1/MotDrvDiagcFltChk/MeasdPhaFltChkABC/NtcStInfoPhaC/DetermineBitsetC/BitsetStsC/Copyright1 ==

== system ES320A_MotDrvDiagc/MotDrvDiagc/MotDrvDiagcPer1/MotDrvDiagcFltChk/MeasdPhaFltChkABC/NtcStInfoPhaC/DetermineBitsetC/BitsetStsC1/Copyright1 ==

== system ES320A_MotDrvDiagc/MotDrvDiagc/MotDrvDiagcPer1/MotDrvDiagcFltChk/MeasdPhaFltChkDEF/NtcStInfoPhaD/DetermineBitsetD/BitsetStsD/Copyright1 ==

== system ES320A_MotDrvDiagc/MotDrvDiagc/MotDrvDiagcPer1/MotDrvDiagcFltChk/MeasdPhaFltChkDEF/NtcStInfoPhaD/DetermineBitsetD/BitsetStsD1/Copyright1 ==

== system ES320A_MotDrvDiagc/MotDrvDiagc/MotDrvDiagcPer1/MotDrvDiagcFltChk/MeasdPhaFltChkDEF/NtcStInfoPhaE/DetermineBitsetE/BitsetStsE/Copyright1 ==

== system ES320A_MotDrvDiagc/MotDrvDiagc/MotDrvDiagcPer1/MotDrvDiagcFltChk/MeasdPhaFltChkDEF/NtcStInfoPhaE/DetermineBitsetE/BitsetStsE1/Copyright1 ==

== system ES320A_MotDrvDiagc/MotDrvDiagc/MotDrvDiagcPer1/MotDrvDiagcFltChk/MeasdPhaFltChkDEF/NtcStInfoPhaF/DetermineBitsetF/BitsetStsF/Copyright1 ==

== system ES320A_MotDrvDiagc/MotDrvDiagc/MotDrvDiagcPer1/MotDrvDiagcFltChk/MeasdPhaFltChkDEF/NtcStInfoPhaF/DetermineBitsetF/BitsetStsF1/Copyright1 ==
